simulink model "buck_converter_VMC_soft_feedforward"  (R2021a)
settings: Solver=VariableStepAuto  StartTime=0.0  StopTime=t_sim  RelTol=1e-3
values from neighbouring files (symbols this model uses):
  C = 600e-6    (= 0.0006)    [boost_parameters.m]    (also in buck_parameters.m = 0.0002)
  iL_0 = 0    [boost_parameters.m]    (also in buck_parameters.m)
  K_d = 0.04    [soft_start.m]    (also in soft_start_feedforward_backward.m; without_soft_start.m)
  K_i = 200000    [soft_start.m]    (also in soft_start_feedforward_backward.m; without_soft_start.m)
  K_p = 30    [soft_start.m]    (also in soft_start_feedforward_backward.m; without_soft_start.m)
  L = 50e-6    (= 5e-05)    [boost_parameters.m]    (also in buck_parameters.m = 5e-07)
  R = 1    [boost_parameters.m]    (also in buck_parameters.m; small_signal_model.m = 10; soft_start.m; soft_start_feedforward_backward.m)
  r_1 = 5e-3    (= 0.005)    [boost_parameters.m]    (also in buck_parameters.m)
  r_2 = 5e-3    (= 0.005)    [boost_parameters.m]    (also in buck_parameters.m)
  r_C = 3e-3    (= 0.003)    [boost_parameters.m]    (also in buck_parameters.m)
  r_L = 5e-3    (= 0.005)    [boost_parameters.m]    (also in buck_parameters.m)
  T = 2e-6    (= 2e-06)    [boost_parameters.m]    (also in buck_parameters.m)
  t_slew = 0.1e-3    (= 0.0001)    [soft_start.m]    (also in soft_start_feedforward_backward.m; without_soft_start.m)
  T_transient = 0.5    [soft_start.m]    (also in soft_start_feedforward_backward.m = 0.0005; without_soft_start.m = 0.0005)
  V_m = 10    [small_signal_model.m]    (also in soft_start.m; soft_start_feedforward_backward.m; without_soft_start.m)
  vC_0 = 0    [boost_parameters.m]    (also in buck_parameters.m)
  Vin = 12    [boost_parameters.m]    (also in buck_parameters.m; small_signal_model.m)
  Vref = 24    [boost_parameters.m]    (also in buck_parameters.m = 1.2; small_signal_model.m = 1.2)
  Vtrans = 0    [soft_start.m]    (also in soft_start_feedforward_backward.m = 6; without_soft_start.m = 6)
libraries: simulink x2, pid_lib x1, simulink_extras x1
settings Model: Creator=Hari Prasad Adhikari  LastModifiedBy=Hari Prasad Adhikari

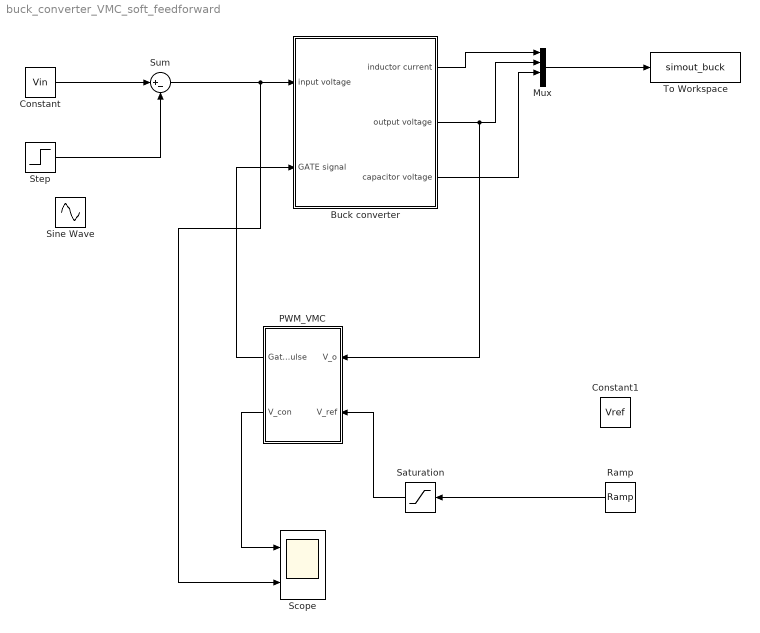
== system buck_converter_VMC_soft_feedforward ==
  Buck converter : Subsystem
  Constant : Constant  Value=Vin
  Constant1 : Constant  Value=Vref
  Mux : Mux
  PWM_VMC : Subsystem
  Ramp : simulink/Sources/Ramp  slope=Vref/t_slew  start=0  InitialOutput=0
  Saturation : Saturate  UpperLimit=Vref  LowerLimit=0
  Scope : Scope  NumInputPorts=2
  Sine Wave : Sin  Amplitude=3  Frequency=2*pi*1e3  SampleTime=0
  Step : Step  Time=T_transient  After=Vtrans  SampleTime=0
  Sum : Sum  Inputs=|+-
  To Workspace : ToWorkspace  VariableName=simout_buck  SaveFormat=Timeseries  SampleTime=-1
  wires:
  Buck converter/1(inductor current) -> Mux/1
  Buck converter/2(output voltage) -> Mux/2, PWM_VMC/1(V_o)
  Buck converter/3(capacitor voltage) -> Mux/3
  Mux/1 -> To Workspace/1
  PWM_VMC/1(Gate Pulse) -> Buck converter/2(GATE signal)
  Ramp/1 -> Saturation/1
  PWM_VMC/2(V_con) -> Scope/1
  Constant/1 -> Sum/1
  Sum/1 -> Scope/2, Buck converter/1(input voltage)
  Saturation/1 -> PWM_VMC/2(V_ref)
  Step/1 -> Sum/2

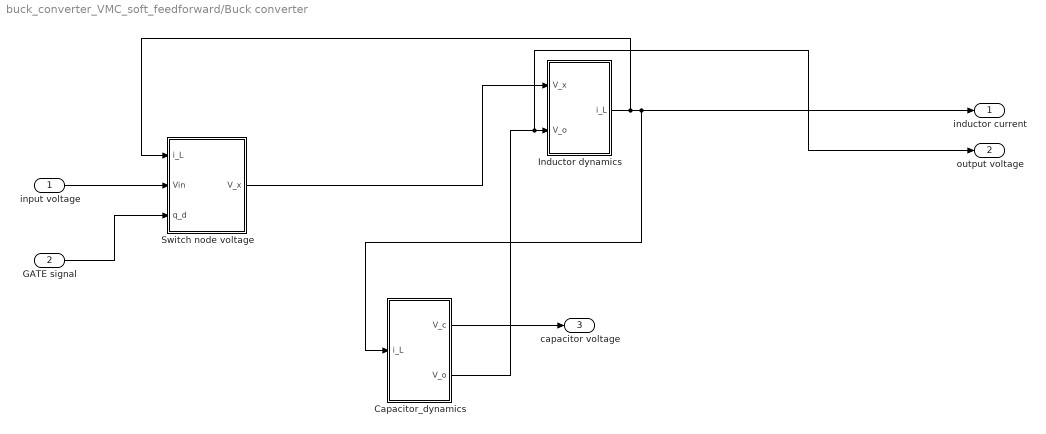
== system buck_converter_VMC_soft_feedforward/Buck converter ==
  input voltage : Inport
  GATE signal : Inport  Port=2
  Capacitor_dynamics : Subsystem
  Inductor dynamics : Subsystem
  Switch node voltage : Subsystem
  inductor current : Outport
  output voltage : Outport  Port=2
  capacitor voltage : Outport  Port=3
  wires:
  Capacitor_dynamics/1(V_c) -> capacitor voltage/1
  Inductor dynamics/1(i_L) -> inductor current/1, Capacitor_dynamics/1(i_L), Switch node voltage/1(i_L)
  Capacitor_dynamics/2(V_o) -> output voltage/1, Inductor dynamics/2(V_o)
  Switch node voltage/1(V_x) -> Inductor dynamics/1(V_x)
  GATE signal/1 -> Switch node voltage/3(q_d)
  input voltage/1 -> Switch node voltage/2(Vin)

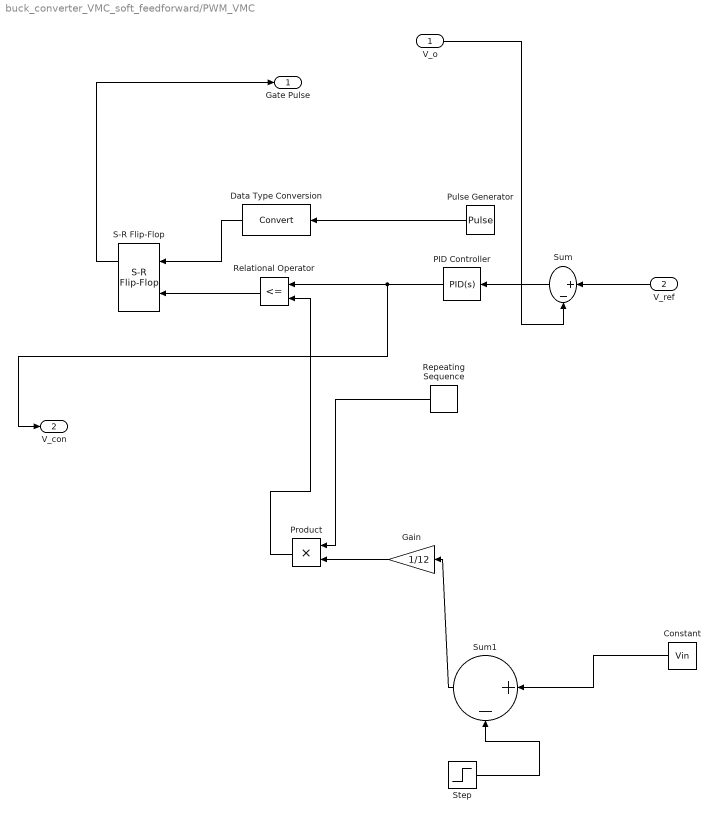
== system buck_converter_VMC_soft_feedforward/PWM_VMC ==
  V_o : Inport
  V_ref : Inport  Port=2
  Constant : Constant  Value=Vin
  Data Type Conversion : DataTypeConversion  OutMin=[0]  OutMax=[1]
  Gain : Gain  Gain=1/12
  PID Controller : pid_lib/PID Controller  Controller=PID  Form=Parallel  TimeDomain=Continuous-time  UseExternalTs=off  SampleTime=-1  IntegratorMethod=Forward Euler  FilterMethod=Forward Euler  ControllerParametersSource=internal  P=K_p  I=K_i  D=K_d  UseFilter=on  N=100  TunerSelectOption=Transfer Function Based (PID Tuner App)  InitialConditionSource=internal  InitialConditionForIntegrator=0  InitialConditionForFilter=0  DifferentiatorICPrevScaledInput=0  ExternalReset=none  TrackingMode=off  Kt=1  LimitOutput=off  SatLimitsSource=internal  UpperSaturationLimit=inf  LowerSaturationLimit=-inf  LinearizeAsGain=on  AntiWindupMode=none  Kb=1  POutMin=[]  POutMax=[]  IOutMin=[]  IOutMax=[]  DOutMin=[]  DOutMax=[]  NOutMin=[]  NOutMax=[]  SumOutMin=[]  SumOutMax=[]  SaturationOutMin=[]  SaturationOutMax=[]  PParamMin=[]  PParamMax=[]  IParamMin=[]  IParamMax=[]  DParamMin=[]  DParamMax=[]  NParamMin=[]  NParamMax=[]  KbParamMin=[]  KbParamMax=[]  KtParamMin=[]  KtParamMax=[]  KbOutMin=[]  KbOutMax=[]  KtOutMin=[]  KtOutMax=[]  IntegratorOutMin=[]  IntegratorOutMax=[]  FilterOutMin=[]  FilterOutMax=[]  SumI1OutMin=[]  SumI1OutMax=[]  SumI2OutMin=[]  SumI2OutMax=[]  SumI3OutMin=[]  SumI3OutMax=[]  SumI4OutMin=[]  SumI4OutMax=[]  SumDOutMin=[]  SumDOutMax=[]  DifferentiatorOutMin=[]  DifferentiatorOutMax=[]  FilterDiffOutCoefMin=[]  FilterDiffOutCoefMax=[]  ReciprocalOutMin=[]  ReciprocalOutMax=[]  SumDenOutMin=[]  SumDenOutMax=[]  SumNumOutMin=[]  SumNumOutMax=[]  DivideOutMin=[]  DivideOutMax=[]  UdiffTsProdOutMin=[]  UdiffTsProdOutMax=[]  NTsProdOutMin=[]  NTsProdOutMax=[]  UintegralTsProdOutMin=[]  UintegralTsProdOutMax=[]  UngainTsProdOutMin=[]  UngainTsProdOutMax=[]  IntegratorContinuousStateAttributes=''  IntegratorStateMustResolveToSignalObject=off  IntegratorRTWStateStorageClass=Auto  FilterContinuousStateAttributes=''  FilterStateMustResolveToSignalObject=off  FilterRTWStateStorageClass=Auto  ParallelPVariant=InternalParameters  IdealPVariant=Disabled  IVariant=InternalParameters  DVariant=InternalParameters  IntegratorVariant=Continuous  SatVariant=Disabled  AWVariant=Passthrough  PCopyVariant=Disabled  TRVariant=Disabled  FdbkBlocksVariant=Forward  IdealPFdbkVariant=Disabled  SatFdbkVariant=Disabled  DerivativeFilterVariant=ContFilter  NVariant=InternalParameters  NCopyVariant=Disabled  FilterICVariant=InternalICsFilter  IntegratorICVariant=InternalICs  ExternalResetVariant=Disabled  TRSumVariant=Passthrough  SumFdbkVariant=Disabled  SumVariant=Sum_PID  TsampFilterVariant=InternalTs  TsampNgainVariant=Passthrough  TsampIntegralVariant=Passthrough  ExternalSaturationOutDataTypeStr=Inherit: Same as second input
  Product : Product
  Pulse Generator : DiscretePulseGenerator  PulseType=Time based  Period=T  PulseWidth=50
  Relational Operator : RelationalOperator  Operator=<=  OutDataTypeStr=boolean  RndMeth=Simplest
  Repeating Sequence : simulink/Sources/Repeating Sequence  rep_seq_t=[0 T]  rep_seq_y=[0 V_m]
  S-R Flip-Flop : simulink_extras/Flip Flops/S-R Flip-Flop  initial_condition=0
  Step : Step  Time=T_transient  After=Vtrans  SampleTime=0
  Sum : Sum  Inputs=|+-
  Sum1 : Sum  Inputs=|+-
  Gate Pulse : Outport
  V_con : Outport  Port=2
  wires:
  Repeating Sequence/1 -> Product/1
  Sum/1 -> PID Controller/1
  Data Type Conversion/1 -> S-R Flip-Flop/1
  Pulse Generator/1 -> Data Type Conversion/1
  V_ref/1 -> Sum/1
  PID Controller/1 -> V_con/1, Relational Operator/1
  Relational Operator/1 -> S-R Flip-Flop/2
  V_o/1 -> Sum/2
  S-R Flip-Flop/1 -> Gate Pulse/1
  Gain/1 -> Product/2
  Sum1/1 -> Gain/1
  Constant/1 -> Sum1/1
  Step/1 -> Sum1/2
  Product/1 -> Relational Operator/2

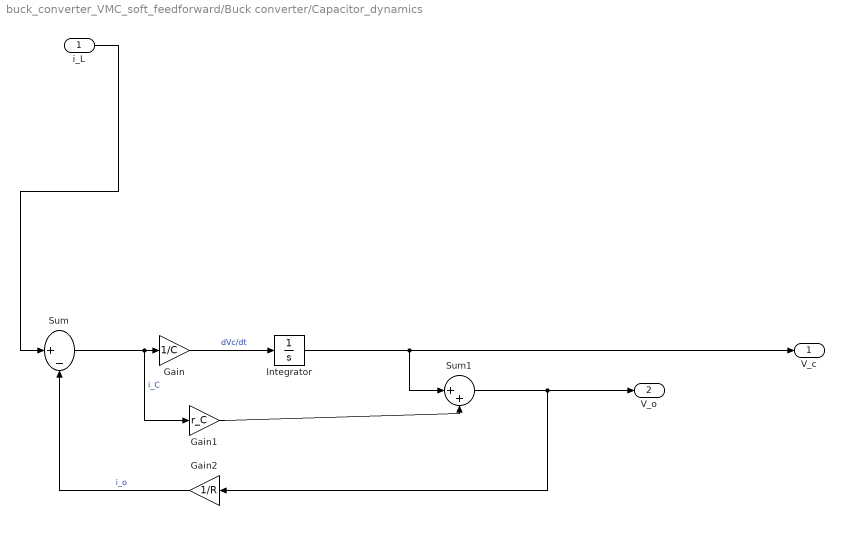
== system buck_converter_VMC_soft_feedforward/Buck converter/Capacitor_dynamics ==
  i_L : Inport
  Gain : Gain  Gain=1/C
  Gain1 : Gain  Gain=r_C
  Gain2 : Gain  Gain=1/R
  Integrator : Integrator  InitialCondition=vC_0
  Sum : Sum  Inputs=|+-
  Sum1 : Sum  Inputs=|++
  V_c : Outport
  V_o : Outport  Port=2
  wires:
  Integrator/1 -> V_c/1, Sum1/1
  Sum1/1 -> V_o/1, Gain2/1
  Gain1/1 -> Sum1/2
  Sum/1 -> Gain1/1, Gain/1  "i_C"
  Gain2/1 -> Sum/2  "i_o"
  Gain/1 -> Integrator/1  "dVc/dt"
  i_L/1 -> Sum/1

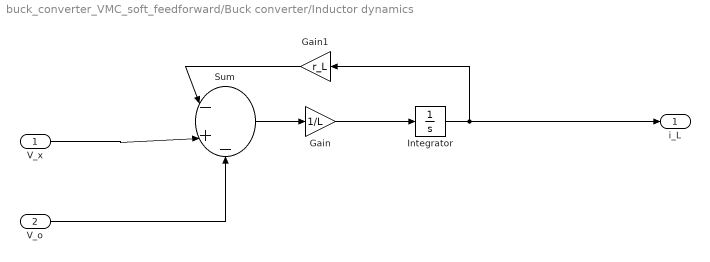
== system buck_converter_VMC_soft_feedforward/Buck converter/Inductor dynamics ==
  V_x : Inport
  V_o : Inport  Port=2
  Gain : Gain  Gain=1/L
  Gain1 : Gain  Gain=r_L
  Integrator : Integrator  InitialCondition=iL_0
  Sum : Sum  Inputs=|-+-
  i_L : Outport
  wires:
  Integrator/1 -> i_L/1, Gain1/1
  Gain/1 -> Integrator/1
  V_o/1 -> Sum/3
  Sum/1 -> Gain/1
  Gain1/1 -> Sum/1
  V_x/1 -> Sum/2

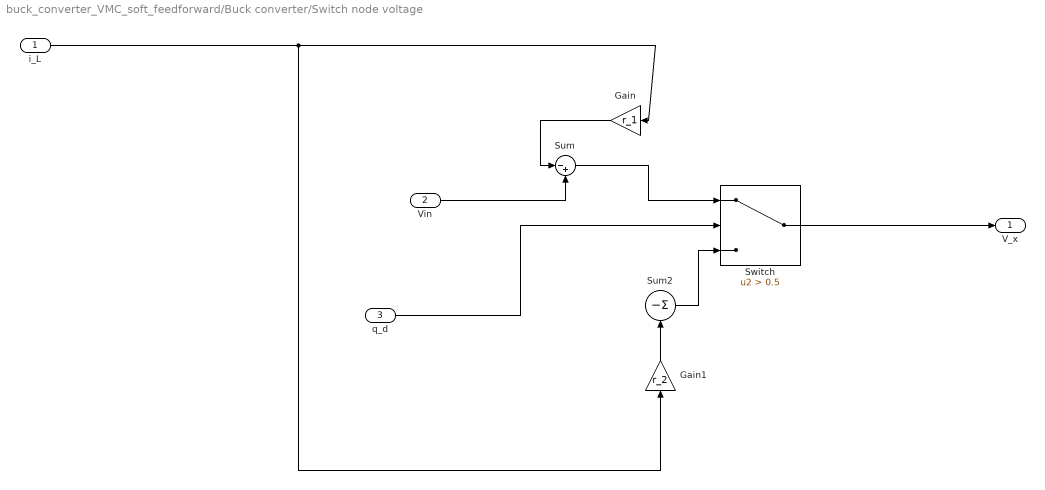
== system buck_converter_VMC_soft_feedforward/Buck converter/Switch node voltage ==
  i_L : Inport
  Vin : Inport  Port=2
  q_d : Inport  Port=3
  Gain : Gain  Gain=r_1
  Gain1 : Gain  Gain=r_2
  Sum : Sum  Inputs=|-+
  Sum2 : Sum  Inputs=|-
  Switch : Switch  Criteria=u2 > Threshold  Threshold=0.5
  V_x : Outport
  wires:
  Gain/1 -> Sum/1
  Gain1/1 -> Sum2/1
  i_L/1 -> Gain1/1, Gain/1
  Switch/1 -> V_x/1
  Sum/1 -> Switch/1
  q_d/1 -> Switch/2
  Sum2/1 -> Switch/3
  Vin/1 -> Sum/2
